simulink model "gi_tract"  (R2024b)
settings: Solver=VariableStepAuto  StartTime=0.0  StopTime=3000  RelTol=1e-3
settings Model: Creator=sunzi  LastModifiedBy=sunzi

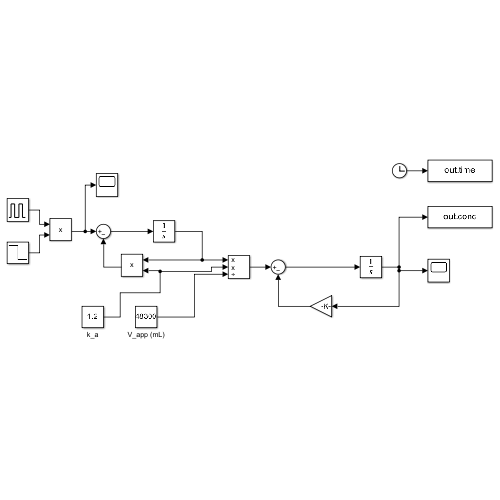
[thumbnail: Simulink's stored preview of the top-level diagram]
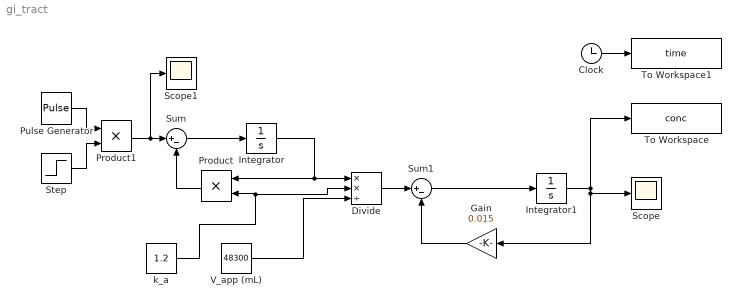
== system gi_tract ==
  Clock : Clock
  Divide : Product  Inputs=**/
  Gain : Gain  Gain=0.015
  Integrator : Integrator
  Integrator1 : Integrator
  Product : Product
  Product1 : Product
  Pulse Generator : DiscretePulseGenerator  PulseType=Time based  Amplitude=14000/5  Period=600  PulseWidth=(5/600)*100
  Scope : Scope
  Scope1 : Scope
  Step : Step  Time=1700  Before=1  After=0  SampleTime=0
  Sum : Sum  Inputs=|+-
  Sum1 : Sum  Inputs=|+-
  To Workspace : ToWorkspace  VariableName=conc  SampleTime=-1
  To Workspace1 : ToWorkspace  VariableName=time  SaveFormat=Timeseries  SampleTime=-1
  V_app (mL) : Constant  Value=48300
  k_a : Constant  Value=1.2
  wires:
  Integrator/1 -> Divide/1, Product/1
  Sum/1 -> Integrator/1
  k_a/1 -> Divide/2, Product/2
  V_app (mL)/1 -> Divide/3
  Gain/1 -> Sum1/2
  Integrator1/1 -> Gain/1, Scope/1, To Workspace/1
  Clock/1 -> To Workspace1/1
  Sum1/1 -> Integrator1/1
  Divide/1 -> Sum1/1
  Product/1 -> Sum/2
  Pulse Generator/1 -> Product1/1
  Product1/1 -> Scope1/1, Sum/1
  Step/1 -> Product1/2
